simulink model "full_order_observer_simulation"  (R2016a)
settings: Solver=VariableStepAuto  StartTime=0.0  StopTime=20.0  RelTol=1e-3
settings Model: Creator=micah  LastModifiedBy=micah

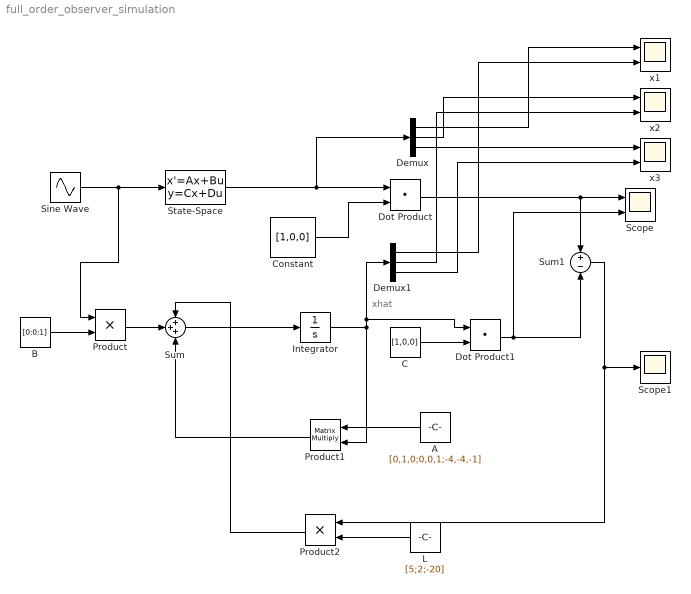
== system full_order_observer_simulation ==
  note: xhat
  A : Constant  Value=[0,1,0;0,0,1;-4,-4,-1]  VectorParams1D=off
  B : Constant  Value=[0;0;1]  VectorParams1D=off
  C : Constant  Value=[1,0,0]  VectorParams1D=off
  Constant : Constant  Value=[1,0,0]
  Demux : Demux  Outputs=3
  Demux1 : Demux  Outputs=3
  Dot Product : DotProduct  InputSameDT=on  OutDataTypeStr=Inherit: Inherit via internal rule
  Dot Product1 : DotProduct  InputSameDT=on  OutDataTypeStr=Inherit: Inherit via internal rule
  Integrator : Integrator  InitialCondition=[0;0;0]
  "L " : Constant  Value=[5;2;-20]
  Product : Product
  Product1 : Product  Multiplication=Matrix(*)
  Product2 : Product
  Scope : Scope  NumInputPorts=2
  Scope1 : Scope
  Sine Wave : Sin  SampleTime=0
  State-Space : StateSpace  A=[0,1,0;0,0,1;-4,-4,-1]  B=[0;0;1]  C=[1,0,0;0,1,0;0,0,1]  D=[0;0;0]  X0=[1,-1,1]
  Sum : Sum  Inputs=+++
  Sum1 : Sum  Inputs=+-
  x1 : Scope  NumInputPorts=2
  x2 : Scope  NumInputPorts=2
  x3 : Scope  NumInputPorts=2
  wires:
  Sine Wave/1 -> Product/1, State-Space/1
  State-Space/1 -> Demux/1, Dot Product/1
  Constant/1 -> Dot Product/2
  Dot Product/1 -> Sum1/1, Scope/1
  B/1 -> Product/2
  Product/1 -> Sum/2
  Sum/1 -> Integrator/1
  A/1 -> Product1/1
  Product1/1 -> Sum/3
  C/1 -> Dot Product1/2
  Dot Product1/1 -> Scope/2, Sum1/2
  Sum1/1 -> Product2/1, Scope1/1
  "L "/1 -> Product2/2
  Product2/1 -> Sum/1
  Demux/1 -> x1/1
  Demux/2 -> x2/1
  Demux/3 -> x3/1
  Integrator/1 -> Dot Product1/1, Demux1/1, Product1/2
  Demux1/1 -> x1/2
  Demux1/2 -> x2/2
  Demux1/3 -> x3/2
